simulink model "Gravity_Well_r2007a"  (Simulink 6.0)
settings: Solver=ode1  StartTime=0.0  StopTime=inf  FixedStep=0.001  RelTol=1e-3
undefined symbols (not defined in the file): HIL, qc_get_step_size
libraries: quarc_library x4, vrlib x1
CloseFcn:
  | rtwprivate ssgencode ModelCloseRequest GravityWell2
settings Model: Creator=PKaram  LastModifiedBy=ajavid  SimulationMode=external  ExtModeTrigDuration=10000
settings SolverCC: PositivePriorityOrder=on
settings OptimizationCC: InlineInvariantSignals=off  ExpressionDepthLimit=2147483647  SimCompilerOptimization=Off
settings DebuggingCC: SignalResolutionControl=UseLocalSettings  FcnCallInpInsideContextMsg=Use local settings  StateNameClashWarn=warning  StrictBusMsg=Warning
settings HardwareCC: TargetHWDeviceType=32-bit Generic
settings RTWCC: SystemTargetFile=quarc_windows.tlc  TemplateMakefile=quarc_default_tmf  Description=QuaRC Win32 Target  ProcessScript=quarc_windows_make_rtw_hook  RTWCompilerOptimization=Off
settings CodeAppCC: CustomSymbolStrType=$N$R$M
settings STFCustomTargetCC: TargetFcnLib=ansi_tfl_tmw.mat  TargetPreCompLibLocation=C:\DOCUME~1\ALLUSE~1\APPLIC~1\QuaRC\lib\2007b\windows\release  GenFloatMathFcnCalls=ANSI_C  SystemTargetFile=quarc_windows.tlc
settings GRTTargetCC: TargetPreCompLibLocation=C:\DOCUME~1\ALLUSE~1\APPLIC~1\QuaRC\lib\2007b\windows\release  CompOptLevelCompliant=off  MatFileLogging=off  ExtMode=on  ExtModeMexFile=quarc_comm

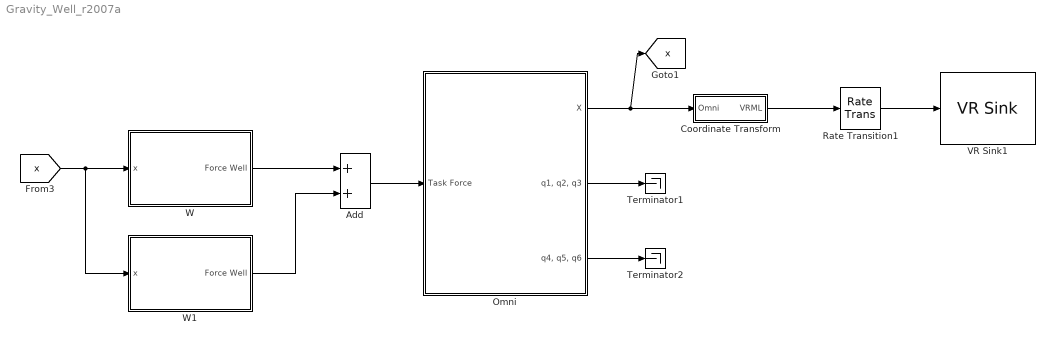
== system Gravity_Well_r2007a ==
  Add : Sum  OutDataType=sfix(16)  OutScaling=2^-10
  Coordinate Transform : Subsystem
  Omni : Subsystem
  Rate Transition1 : RateTransition
  Terminator1 : Terminator
  Terminator2 : Terminator
  VR Sink1 : vrlib/VR Sink  SampleTime=0.1  ViewEnable=on  RemoteChange=off  RemoteView=on  FieldsWritten=Avatar.translation.3.1.double  WorldFileName=GravityWell.txt  AutoView=on  VideoDimensions=[]  FigureProperties="{'Position', 'Name', 'Viewpoint', 'CameraBound', 'CameraDirection', 'CameraPosition', 'CameraUpVector', 'ZoomFactor', 'Antialiasing', 'Headlight', 'Lighting', 'NavPanel', 'StatusBar', 'ToolBar', 'Textures', 'Transparency', 'Wireframe', 'NavZones', 'NavMode', 'NavSpeed', 'Record2DCompressMethod', 'Record2DCompressQuality', 'Record2D', 'Record2DFileName', 'Record2DFPS'; [5.0000000000000000e+000  9.2000000000000000e+001  5.7600000000000000e+002  3.8000000000000000e+002], '', '_untitled_1', 'on', [0.0000000000000000e+000  0.0000000000000000e+000 -1.0000000000000000e+000], [0.0000000000000000e+000  0.0000000000000000e+000  0.0000000000000000e+000], [0.0000000000000000e+000  1.0000000000000000e+000  0.0000000000000000e+000], [1.0000000000000000e+000], 'off', 'on', 'on', 'halfbar', 'off', 'on', 'on', 'on', 'off', 'off', 'fly', 'normal', 'auto', [7.5000000000000000e+001], 'off', '%f_anim_%n.avi', [1.5000000000000000e+001]}"
  W : Subsystem
  W1 : Subsystem
  tag scope: x=global
  wires:
  [x] -> W/1("x "), W1/1("x ")
  Coordinate Transform/1("VRML ") -> Rate Transition1/1
  Rate Transition1/1 -> VR Sink1/1
  W/1(Force Well) -> Add/1
  W1/1(Force Well) -> Add/2
  Add/1 -> Omni/1(Task Force)
  Omni/1(X) -> Coordinate Transform/1(Omni), [x]
  Omni/3("q4, q5, q6") -> Terminator2/1
  Omni/2("q1, q2, q3") -> Terminator1/1

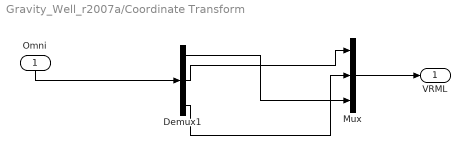
== system Gravity_Well_r2007a/Coordinate Transform ==
  Omni : Inport  Orientation=down
  Demux1 : Demux  Outputs=3
  Mux : Mux  Inputs=3
  "VRML " : Outport
  wires:
  Omni/1 -> Demux1/1
  Mux/1 -> "VRML "/1
  Demux1/1 -> Mux/3
  Demux1/2 -> Mux/1
  Demux1/3 -> Mux/2

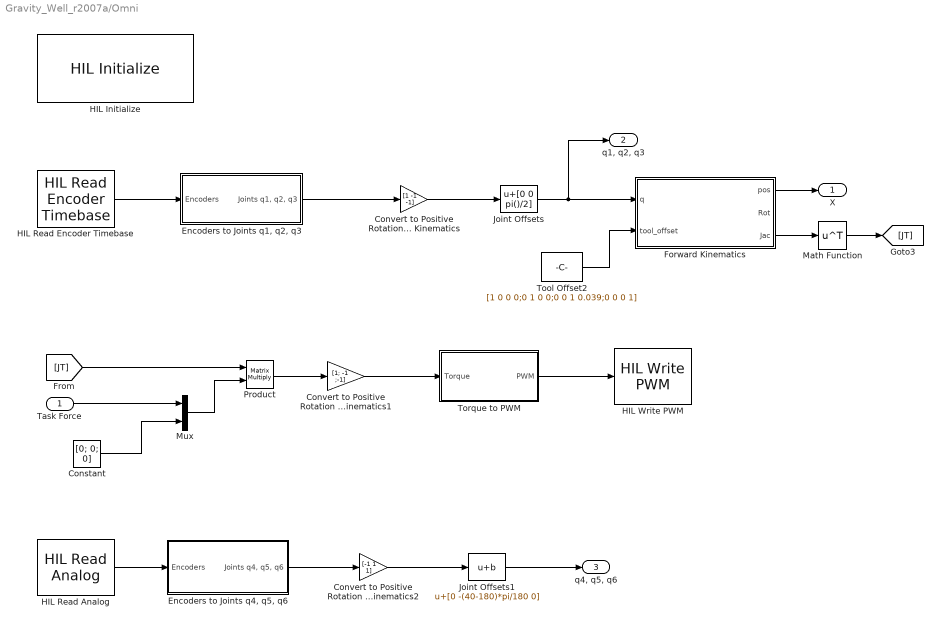
== system Gravity_Well_r2007a/Omni ==
  Task Force : Inport
  Constant : Constant  Value=[0; 0; 0]  VectorParams1D=off  OutDataType=sfix(16)  OutScaling=2^0
  Convert to Positive Rotation Convension Used in Kinematics : Gain  Gain=[1 -1 -1]  ParameterDataType=sfix(16)  ParameterScaling=2^0  OutDataType=sfix(16)  OutScaling=2^0
  Convert to Positive Rotation Convension Used in Kinematics1 : Gain  Gain=[1; -1 ;-1]  ParameterDataType=sfix(16)  ParameterScaling=2^0  OutDataType=sfix(16)  OutScaling=2^0
  Convert to Positive Rotation Convension Used in Kinematics2 : Gain  Gain=[-1 1 1]  ParameterDataType=sfix(16)  ParameterScaling=2^0  OutDataType=sfix(16)  OutScaling=2^0
  "Encoders to Joints q1, q2, q3" : Subsystem
  "Encoders to Joints q4, q5, q6" : Subsystem
  "Forward Kinematics " : Stateflow chart
      settings: PermitHierarchicalResolution=ParametersOnly
  HIL Initialize : quarc_library/Data Acquisition/Generic/Configuration/HIL Initialize  object_name=HIL-1  board_type=phantom_omni  board_number=0  active=on  hardware_clocks=[]  clock_modes=[]  set_clock_params_at_start=off  set_clock_params_at_switch_in=off  analog_input_channels=0:1  analog_input_maximums=10  analog_input_minimums=-10  set_analog_input_params_at_start=off  set_analog_input_params_at_switch_in=off  analog_output_channels=[]  analog_output_maximums=[]  analog_output_minimums=[]  initial_analog_outputs=[]  final_analog_outputs=[]  watchdog_analog_outputs=0  set_analog_output_params_at_start=off  set_analog_output_params_at_switch_in=off  set_analog_outputs_at_start=off  set_analog_outputs_at_switch_in=off  set_analog_outputs_at_terminate=off  set_analog_outputs_at_switch_out=off  set_analog_outputs_on_watchdog=off  digital_input_channels=[]  digital_output_channels=[]  initial_digital_outputs=[]  final_digital_outputs=[]  watchdog_digital_outputs=0  set_digital_outputs_at_start=off  set_digital_outputs_at_switch_in=off  set_digital_outputs_at_terminate=off  set_digital_outputs_at_switch_out=off  set_digital_outputs_on_watchdog=off  encoder_channels=0:2  quadrature=[]  encoder_filter_frequency=[]  initial_encoder_counts=0  set_encoder_params_at_start=off  set_encoder_params_at_switch_in=off  set_encoder_counts_at_start=off  set_encoder_counts_at_switch_in=off  pwm_channels=0:2  pwm_modes=[]  pwm_frequency=[]  initial_pwm_outputs=0  final_pwm_outputs=0  watchdog_pwm_outputs=0  set_pwm_params_at_start=off  set_pwm_params_at_switch_in=off  set_pwm_outputs_at_start=on  set_pwm_outputs_at_switch_in=off  set_pwm_outputs_at_terminate=on  set_pwm_outputs_at_switch_out=off  set_pwm_outputs_on_watchdog=off  other_output_channels=[]  initial_other_outputs=[]  final_other_outputs=[]  watchdog_other_outputs=0  set_other_outputs_at_start=off  set_other_outputs_at_switch_in=off  set_other_outputs_at_terminate=off  set_other_outputs_at_switch_out=off  set_other_outputs_on_watchdog=off
  HIL Read Analog : quarc_library/Data Acquisition/Generic/Immediate I//O/HIL Read Analog  object_name=HIL-1  channels=[0:2]  sample_time=qc_get_step_size  active=on  vector_output=on
  HIL Read Encoder Timebase : quarc_library/Data Acquisition/Generic/Timebases/HIL Read Encoder Timebase  object_name=HIL-1  clock=0  channels=0:2  samples_in_buffer=max(ceil(1/qc_get_step_size), 1)  active=on  vector_output=on  data_type_mode=Inherit via back propagation  data_type=double
  HIL Write PWM : quarc_library/Data Acquisition/Generic/Immediate I//O/HIL Write PWM  object_name=HIL-1  channels=0:2  sample_time=-1  active=off  vector_input=on
      settings: AttributesFormatString=(%<object_name>)
  Joint Offsets : Bias  Bias=[0 0 pi()/2]
  Joint Offsets1 : Bias  Bias=[0 -(40-180)*pi/180 0]  SaturateOnIntegerOverflow=on
  Math Function : Math  Operator=transpose  OutDataType=sfix(16)  OutScaling=2^0  SaturateOnIntegerOverflow=on
  Mux : Mux  Inputs=2
  Product : Product  Multiplication=Matrix(*)  OutDataType=sfix(16)  OutScaling=2^0  RndMeth=Zero
  Tool Offset2 : Constant  Value=[1 0 0 0;0 1 0 0;0 0 1 0.039;0 0 0 1]  VectorParams1D=off  OutDataType=sfix(16)  OutScaling=2^0
  Torque to PWM : Subsystem
  X : Outport
  "q1, q2, q3" : Outport  Port=2
  "q4, q5, q6" : Outport  Port=3
  wires:
  Tool Offset2/1 -> "Forward Kinematics "/2(tool_offset)
  Math Function/1 -> [JT]
  "Forward Kinematics "/3(Jac) -> Math Function/1
  [JT] -> Product/1
  Torque to PWM/1(PWM) -> HIL Write PWM/1
  "Forward Kinematics "/1(pos) -> X/1
  Constant/1 -> Mux/2
  Task Force/1 -> Mux/1
  Mux/1 -> Product/2
  "Encoders to Joints q1, q2, q3"/1("Joints q1, q2, q3") -> Convert to Positive Rotation Convension Used in Kinematics/1
  Convert to Positive Rotation Convension Used in Kinematics/1 -> Joint Offsets/1
  Convert to Positive Rotation Convension Used in Kinematics1/1 -> Torque to PWM/1(Torque)
  Product/1 -> Convert to Positive Rotation Convension Used in Kinematics1/1
  Joint Offsets/1 -> "Forward Kinematics "/1(q), "q1, q2, q3"/1
  HIL Read Encoder Timebase/1 -> "Encoders to Joints q1, q2, q3"/1(Encoders)
  HIL Read Analog/1 -> "Encoders to Joints q4, q5, q6"/1(Encoders)
  Convert to Positive Rotation Convension Used in Kinematics2/1 -> Joint Offsets1/1
  "Encoders to Joints q4, q5, q6"/1("Joints q4, q5, q6") -> Convert to Positive Rotation Convension Used in Kinematics2/1
  Joint Offsets1/1 -> "q4, q5, q6"/1

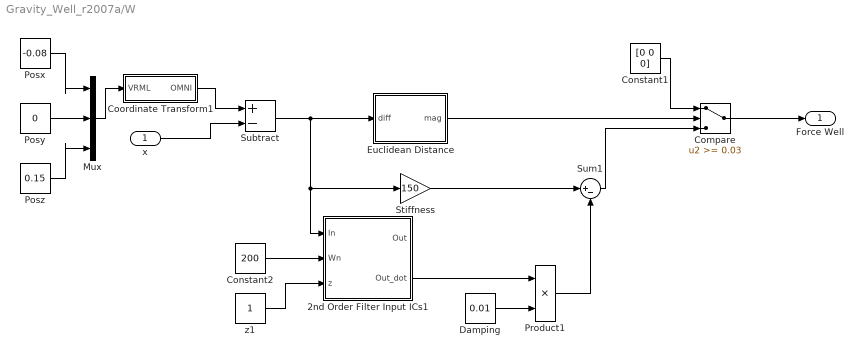
== system Gravity_Well_r2007a/W ==
  "x " : Inport  OutDataType=sfix(16)  OutScaling=2^0
  2nd Order Filter Input ICs1 : Subsystem
  Compare : Switch  Threshold=0.03
  Constant1 : Constant  Value=[0 0 0]  OutDataType=sfix(16)  OutScaling=2^0
  Constant2 : Constant  Value=200  OutDataType=sfix(16)  OutScaling=2^0
  Coordinate Transform1 : Subsystem
  Damping : Constant  Value=0.01  OutDataType=sfix(16)  OutScaling=2^0
  Euclidean Distance : Stateflow chart
      settings: PermitHierarchicalResolution=ParametersOnly
  Mux : Mux  Inputs=3
  Posx : Constant  Value=-0.08  OutDataType=sfix(16)  OutScaling=2^0
  Posy : Constant  Value=0  OutDataType=sfix(16)  OutScaling=2^0
  Posz : Constant  Value=0.15  OutDataType=sfix(16)  OutScaling=2^0
  Product1 : Product  OutDataType=sfix(16)  OutScaling=2^0  RndMeth=Zero
  Stiffness : Gain  Gain=150  ParameterDataType=sfix(16)  ParameterScaling=2^0  OutDataType=sfix(16)  OutScaling=2^0
  Subtract : Sum  Inputs=+-  OutDataType=sfix(16)  OutScaling=2^-10
  Sum1 : Sum  Inputs=|+-  OutDataType=sfix(16)  OutScaling=2^0
  z1 : Constant  OutDataType=sfix(16)  OutScaling=2^0
  Force Well : Outport  OutDataType=sfix(16)  OutScaling=2^0
  wires:
  Coordinate Transform1/1("OMNI ") -> Subtract/1
  z1/1 -> 2nd Order Filter Input ICs1/3(z)
  Constant2/1 -> 2nd Order Filter Input ICs1/2(Wn)
  2nd Order Filter Input ICs1/2(Out_dot) -> Product1/1
  Sum1/1 -> Compare/3
  Product1/1 -> Sum1/2
  Damping/1 -> Product1/2
  Stiffness/1 -> Sum1/1
  "x "/1 -> Subtract/2
  Compare/1 -> Force Well/1
  Constant1/1 -> Compare/1
  Euclidean Distance/1(mag) -> Compare/2
  Subtract/1 -> 2nd Order Filter Input ICs1/1(In), Stiffness/1, Euclidean Distance/1(diff)
  Posx/1 -> Mux/1
  Mux/1 -> Coordinate Transform1/1(VRML)
  Posy/1 -> Mux/2
  Posz/1 -> Mux/3

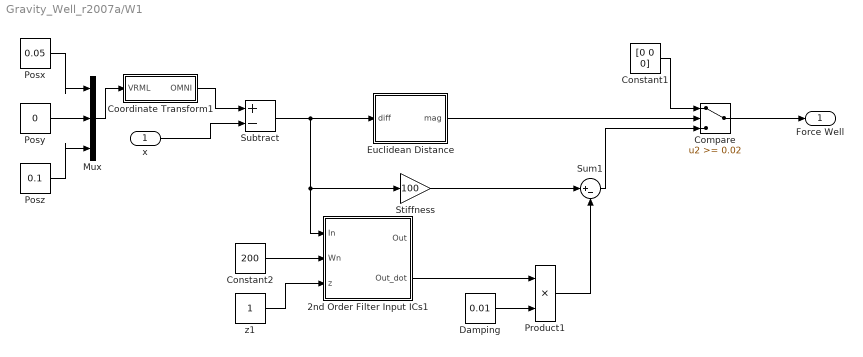
== system Gravity_Well_r2007a/W1 ==
  "x " : Inport  OutDataType=sfix(16)  OutScaling=2^0
  2nd Order Filter Input ICs1 : Subsystem
  Compare : Switch  Threshold=0.02
  Constant1 : Constant  Value=[0 0 0]  OutDataType=sfix(16)  OutScaling=2^0
  Constant2 : Constant  Value=200  OutDataType=sfix(16)  OutScaling=2^0
  Coordinate Transform1 : Subsystem
  Damping : Constant  Value=0.01  OutDataType=sfix(16)  OutScaling=2^0
  Euclidean Distance : Stateflow chart
      settings: PermitHierarchicalResolution=ParametersOnly
  Mux : Mux  Inputs=3
  Posx : Constant  Value=0.05  OutDataType=sfix(16)  OutScaling=2^0
  Posy : Constant  Value=0  OutDataType=sfix(16)  OutScaling=2^0
  Posz : Constant  Value=0.1  OutDataType=sfix(16)  OutScaling=2^0
  Product1 : Product  OutDataType=sfix(16)  OutScaling=2^0  RndMeth=Zero
  Stiffness : Gain  Gain=100  ParameterDataType=sfix(16)  ParameterScaling=2^0  OutDataType=sfix(16)  OutScaling=2^0
  Subtract : Sum  Inputs=+-  OutDataType=sfix(16)  OutScaling=2^-10
  Sum1 : Sum  Inputs=|+-  OutDataType=sfix(16)  OutScaling=2^0
  z1 : Constant  OutDataType=sfix(16)  OutScaling=2^0
  Force Well : Outport  OutDataType=sfix(16)  OutScaling=2^0
  wires:
  Posz/1 -> Mux/3
  Posy/1 -> Mux/2
  Mux/1 -> Coordinate Transform1/1(VRML)
  Posx/1 -> Mux/1
  Subtract/1 -> Euclidean Distance/1(diff), Stiffness/1, 2nd Order Filter Input ICs1/1(In)
  Euclidean Distance/1(mag) -> Compare/2
  Constant1/1 -> Compare/1
  Compare/1 -> Force Well/1
  "x "/1 -> Subtract/2
  Stiffness/1 -> Sum1/1
  Damping/1 -> Product1/2
  Product1/1 -> Sum1/2
  Sum1/1 -> Compare/3
  2nd Order Filter Input ICs1/2(Out_dot) -> Product1/1
  Constant2/1 -> 2nd Order Filter Input ICs1/2(Wn)
  z1/1 -> 2nd Order Filter Input ICs1/3(z)
  Coordinate Transform1/1("OMNI ") -> Subtract/1

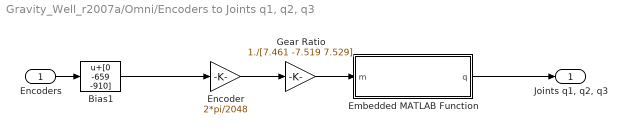
== system Gravity_Well_r2007a/Omni/Encoders to Joints q1, q2, q3 ==
  Encoders : Inport
  Bias1 : Bias  Bias=[0 -659 -910]
  Embedded MATLAB Function : Stateflow chart
      settings: PermitHierarchicalResolution=ParametersOnly
  Encoder : Gain  Gain=2*pi/2048  ParameterDataType=sfix(16)  ParameterScaling=2^0  OutDataType=sfix(16)  OutScaling=2^0
  Gear Ratio : Gain  Gain=1./[7.461 -7.519 7.529]  ParameterDataType=sfix(16)  ParameterScaling=2^0  OutDataType=sfix(16)  OutScaling=2^0
  "Joints q1, q2, q3" : Outport
  wires:
  Embedded MATLAB Function/1(q) -> "Joints q1, q2, q3"/1
  Encoders/1 -> Bias1/1
  Encoder/1 -> Gear Ratio/1
  Gear Ratio/1 -> Embedded MATLAB Function/1(m)
  Bias1/1 -> Encoder/1

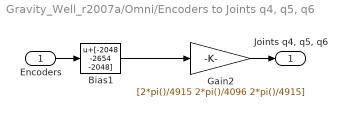
== system Gravity_Well_r2007a/Omni/Encoders to Joints q4, q5, q6 ==
  Encoders : Inport
  Bias1 : Bias  Bias=[-2048 -2654 -2048]
  Gain2 : Gain  Gain=[2*pi()/4915 2*pi()/4096 2*pi()/4915]  ParameterDataType=sfix(16)  ParameterScaling=2^0  OutDataType=sfix(16)  OutScaling=2^0
  "Joints q4, q5, q6" : Outport
  wires:
  Bias1/1 -> Gain2/1
  Encoders/1 -> Bias1/1
  Gain2/1 -> "Joints q4, q5, q6"/1

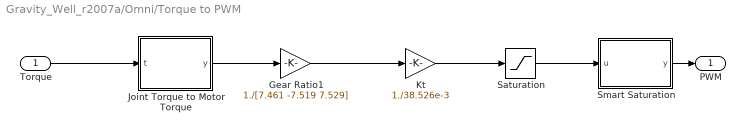
== system Gravity_Well_r2007a/Omni/Torque to PWM ==
  Torque : Inport
  Gear Ratio1 : Gain  Gain=1./[7.461 -7.519 7.529]  ParameterDataType=sfix(16)  ParameterScaling=2^0  OutDataType=sfix(16)  OutScaling=2^0
  Joint Torque to Motor Torque : Stateflow chart
      settings: PermitHierarchicalResolution=ParametersOnly
  Kt : Gain  Gain=1./38.526e-3  ParameterDataType=sfix(16)  ParameterScaling=2^0  OutDataType=sfix(16)  OutScaling=2^0
  Saturation : Saturate  UpperLimit=1.6  LowerLimit=-1.6
  Smart Saturation : Stateflow chart
      settings: PermitHierarchicalResolution=ParametersOnly
  PWM : Outport
  wires:
  Torque/1 -> Joint Torque to Motor Torque/1(t)
  Smart Saturation/1(y) -> PWM/1
  Saturation/1 -> Smart Saturation/1(u)
  Kt/1 -> Saturation/1
  Gear Ratio1/1 -> Kt/1
  Joint Torque to Motor Torque/1(y) -> Gear Ratio1/1

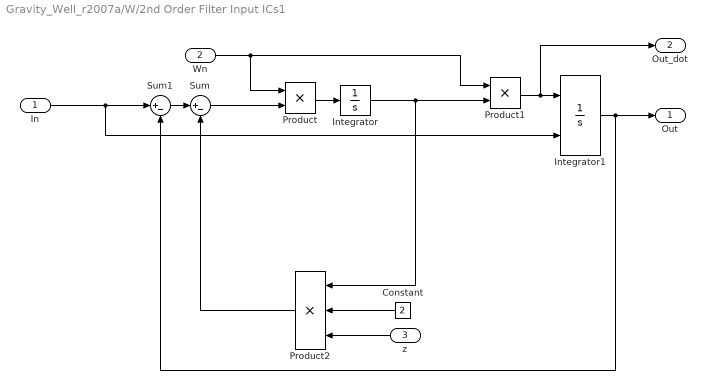
== system Gravity_Well_r2007a/W/2nd Order Filter Input ICs1 ==
  In : Inport  OutDataType=sfix(16)  OutScaling=2^0
  Wn : Inport  Port=2  OutDataType=sfix(16)  OutScaling=2^0
  z : Inport  Orientation=left  Port=3  OutDataType=sfix(16)  OutScaling=2^0
  Constant : Constant  Orientation=left  Value=2  OutDataType=sfix(16)  OutScaling=2^0
  Integrator : Integrator
  Integrator1 : Integrator  InitialConditionSource=external
  Product : Product  OutDataType=sfix(16)  OutScaling=2^0  RndMeth=Zero
  Product1 : Product  OutDataType=sfix(16)  OutScaling=2^0  RndMeth=Zero
  Product2 : Product  Orientation=left  Inputs=3  OutDataType=sfix(16)  OutScaling=2^0  RndMeth=Zero
  Sum : Sum  Inputs=|+-  OutDataType=sfix(16)  OutScaling=2^0
  Sum1 : Sum  Inputs=|+-  OutDataType=sfix(16)  OutScaling=2^0
  Out : Outport  OutDataType=sfix(16)  OutScaling=2^0
  Out_dot : Outport  Port=2  OutDataType=sfix(16)  OutScaling=2^0
  wires:
  Constant/1 -> Product2/2
  z/1 -> Product2/3
  Product2/1 -> Sum/2
  In/1 -> Integrator1/2, Sum1/1
  Sum1/1 -> Sum/1
  Integrator1/1 -> Out/1, Sum1/2
  Integrator/1 -> Product2/1, Product1/2
  Product1/1 -> Out_dot/1, Integrator1/1
  Wn/1 -> Product1/1, Product/1
  Sum/1 -> Product/2
  Product/1 -> Integrator/1

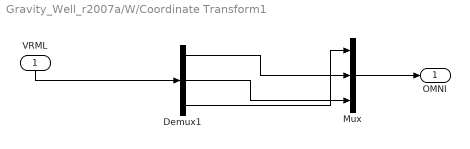
== system Gravity_Well_r2007a/W/Coordinate Transform1 ==
  VRML : Inport  Orientation=down
  Demux1 : Demux  Outputs=3
  Mux : Mux  Inputs=3
  "OMNI " : Outport
  wires:
  Demux1/3 -> Mux/1
  Demux1/2 -> Mux/3
  Demux1/1 -> Mux/2
  Mux/1 -> "OMNI "/1
  VRML/1 -> Demux1/1

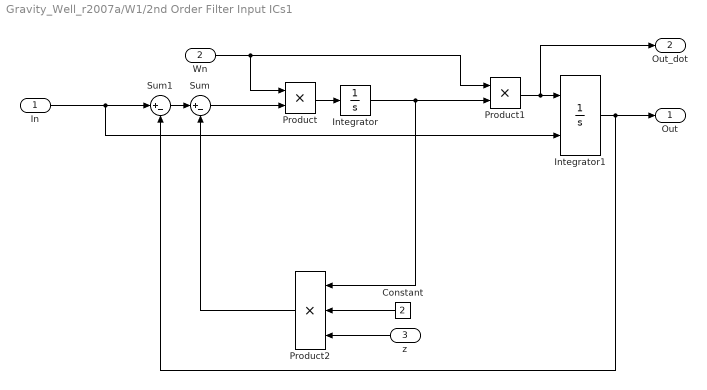
== system Gravity_Well_r2007a/W1/2nd Order Filter Input ICs1 ==
  In : Inport  OutDataType=sfix(16)  OutScaling=2^0
  Wn : Inport  Port=2  OutDataType=sfix(16)  OutScaling=2^0
  z : Inport  Orientation=left  Port=3  OutDataType=sfix(16)  OutScaling=2^0
  Constant : Constant  Orientation=left  Value=2  OutDataType=sfix(16)  OutScaling=2^0
  Integrator : Integrator
  Integrator1 : Integrator  InitialConditionSource=external
  Product : Product  OutDataType=sfix(16)  OutScaling=2^0  RndMeth=Zero
  Product1 : Product  OutDataType=sfix(16)  OutScaling=2^0  RndMeth=Zero
  Product2 : Product  Orientation=left  Inputs=3  OutDataType=sfix(16)  OutScaling=2^0  RndMeth=Zero
  Sum : Sum  Inputs=|+-  OutDataType=sfix(16)  OutScaling=2^0
  Sum1 : Sum  Inputs=|+-  OutDataType=sfix(16)  OutScaling=2^0
  Out : Outport  OutDataType=sfix(16)  OutScaling=2^0
  Out_dot : Outport  Port=2  OutDataType=sfix(16)  OutScaling=2^0
  wires:
  Constant/1 -> Product2/2
  z/1 -> Product2/3
  Product2/1 -> Sum/2
  In/1 -> Integrator1/2, Sum1/1
  Sum1/1 -> Sum/1
  Integrator1/1 -> Out/1, Sum1/2
  Integrator/1 -> Product2/1, Product1/2
  Product1/1 -> Out_dot/1, Integrator1/1
  Wn/1 -> Product1/1, Product/1
  Sum/1 -> Product/2
  Product/1 -> Integrator/1

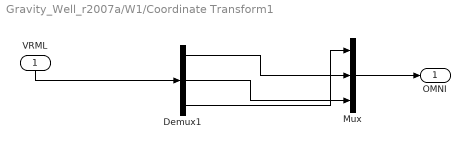
== system Gravity_Well_r2007a/W1/Coordinate Transform1 ==
  VRML : Inport  Orientation=down
  Demux1 : Demux  Outputs=3
  Mux : Mux  Inputs=3
  "OMNI " : Outport
  wires:
  VRML/1 -> Demux1/1
  Mux/1 -> "OMNI "/1
  Demux1/1 -> Mux/2
  Demux1/2 -> Mux/3
  Demux1/3 -> Mux/1

== matlab function W1/Euclidean Distance ==
  data: diff input inherited; mag output inherited
function mag = fcn(diff)
% This block supports the Embedded MATLAB subset.
% See the help menu for details. 

mag = sqrt(diff(1)^2+diff(2)^2+diff(3)^2);

== matlab function Omni/Torque to PWM/Smart Saturation ==
  data: u input inherited; y output inherited size=3
function y = fcn(u)
% Smart Saturation: allows channels to go up to 1.6A 
% unless the total exceeds 2.2A in which case all channels
% are scaled so that the cumulative current is equal to 2.2A.

y = zeros(3,1);
MAX_CURRENT = 2.2; % Define the maximum cumulative current here

total = sum(abs(u));
if (total > MAX_CURRENT)
    y = MAX_CURRENT/total*u;
else
    y = u;
end

== matlab function Omni/Torque to PWM/Joint Torque to Motor Torque ==
  data: t input inherited; y output inherited
function y = fcn( t)
% Smart Saturation: allows channels to go up to 1.6A 
% unless the total exceeds 2.2A in which case all channels
% are scaled so that the cumulative current is equal to 2.2A.
y=[0 0 0]'

y(1)=t(1);
y(3)=t(3);
y(2)=t(2)-t(3);


end

== matlab function Omni/Forward Kinematics  ==
  data: pos output inherited; q input inherited; Rot output inherited; tool_offset input inherited; Jac output inherited
function [pos,Rot,Jac]    = fcn(q,tool_offset)
% This block supports the Embedded MATLAB subset.
% See the help menu for details. 

% Link lengths
L1 = .132;
L2 = .132;

%Define A-matrices
%A1= DH(a_i ,alpha_i    ,d_i    ,theta_i)
A1 = DH(0   ,-pi()/2    ,0      ,q(1));
A2 = DH(L1  ,0          ,0      ,q(2));
A3 = DH(L2   ,0     ,0     ,q(3)-pi/2);

%Define T Matrices
T01=A1;
T02=T01*A2;
T03=T02*A3;

%Axes of rotation in base coordinates. 

z0=[0 0 1]';
z1=T01(1:3,3);
z2=T02(1:3,3);

%Coordinate Frame origins in Base frame coordinates

p0=[0 0 0]';
p1=T01(1:3,4);
p2=T02(1:3,4);
p3=T03(1:3,4);


%tool_offset given with respect to frame 3.
T_tool=T03*tool_offset;
Rot=T03(1:3,1:3);
pos=T_tool(1:3,4);

%Formulation of the Jacobian

%%%%%%%%%%%%%%%%%%%%%%%%%%%%JACOBIAN%%%%%%%%%%%%%%%%%%%%%%%%
Jac = [cross(z0,(pos-p0)) cross(z1,(pos-p1)) cross(z2,(pos-p2))
    z0 z1 z2];

end

function A = DH(a_x, alpha_x, d_z, theta_z)

A_R_z = [cos(theta_z) -sin(theta_z) 0 0;
         sin(theta_z) cos(theta_z) 0 0;
         0 0 1 0;
         0 0 0 1];

A_T_z = [1 0 0 0;
         0 1 0 0;
         0 0 1 d_z;
         0 0 0 1];
     
  

A_T_x = [1 0 0 a_x;
         0 1 0 0;
         0 0 1 0;
         0 0 0 1];

A_R_x = [1 0 0 0;
         0 cos(alpha_x) -sin(alpha_x)  0;
         0 sin(alpha_x) cos(alpha_x) 0;
         0 0 0 1];

A = A_R_z*A_T_z*A_T_x*A_R_x;

end

== matlab function W/Euclidean Distance ==
  data: diff input inherited; mag output inherited
function mag = fcn(diff)
% This block supports the Embedded MATLAB subset.
% See the help menu for details. 

mag = sqrt(diff(1)^2+diff(2)^2+diff(3)^2);

== matlab function Omni/Encoders to Joints q1, q2, q3/Embedded MATLAB Function ==
  data: m input inherited; q output inherited
function q = Motors_2_Joints(m)
q = m;
q(1) = m(1);
q(2) = m(2);
q(3) = m(3) - m(2) -pi/2;
end
